simulink model "FSK_MODEM_v2"  (R2021b)
settings: Solver=VariableStepAuto  StartTime=0.0  StopTime=0.05  RelTol=1e-3
values from neighbouring files (symbols this model uses):
  fcarrier = 10000    [run_modem.m]
  fdelta = (fcarrier/100)*50    (= 5000)    [run_modem.m]
libraries: dsparch4 x5, dspsrcs4 x2, commrandsrc3 x1
settings Model: Creator=caccolillo  LastModifiedBy=caccolillo

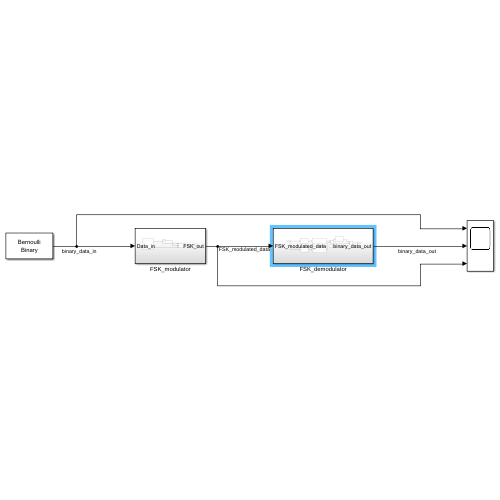
[thumbnail: Simulink's stored preview of the top-level diagram]
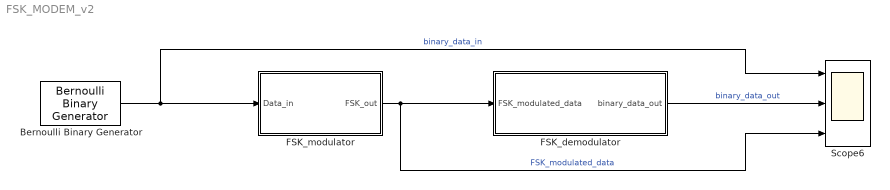
== system FSK_MODEM_v2 ==
  Bernoulli Binary Generator : commrandsrc3/Bernoulli Binary Generator  ProbabilityOfZero=0.5  SeedSource=Auto  Seed=0  SampleTime=20/fcarrier  SamplesPerFrame=1  OutputDataType=double  SimulateUsing=Interpreted execution
  FSK_demodulator : Subsystem
  FSK_modulator : Subsystem
  Scope6 : Scope  NumInputPorts=3
  wires:
  Bernoulli Binary Generator/1 -> FSK_modulator/1(Data_in), Scope6/1  "binary_data_in"
  FSK_demodulator/1(binary_data_out) -> Scope6/2  "binary_data_out"
  FSK_modulator/1(FSK_out) -> Scope6/3, FSK_demodulator/1(FSK_modulated_data)  "FSK_modulated_data"

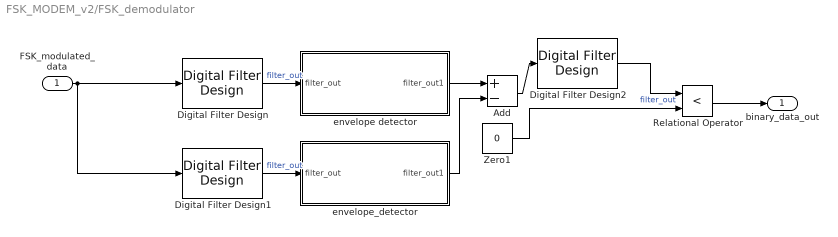
== system FSK_MODEM_v2/FSK_demodulator ==
  FSK_modulated_data : Inport
  Add : Sum  Inputs=+-
  Digital Filter Design : dsparch4/Digital Filter Design  mwdsp_browser_bugfix_var=off
  Digital Filter Design1 : dsparch4/Digital Filter Design  mwdsp_browser_bugfix_var=off
  Digital Filter Design2 : dsparch4/Digital Filter Design  mwdsp_browser_bugfix_var=off
  Relational Operator : RelationalOperator  Operator=<  OutDataTypeStr=boolean  RndMeth=Simplest
  Zero1 : Constant  Value=0  SampleTime=1/(100*fcarrier)
  envelope detector : Subsystem
  envelope_detector : Subsystem
  binary_data_out : Outport
  wires:
  FSK_modulated_data/1 -> Digital Filter Design/1, Digital Filter Design1/1
  Add/1 -> Digital Filter Design2/1
  Digital Filter Design/1 -> envelope detector/1(filter_out)  "filter_out"
  Relational Operator/1 -> binary_data_out/1
  Zero1/1 -> Relational Operator/2
  envelope detector/1(filter_out1) -> Add/1
  envelope_detector/1(filter_out1) -> Add/2
  Digital Filter Design1/1 -> envelope_detector/1(filter_out)  "filter_out"
  Digital Filter Design2/1 -> Relational Operator/1  "filter_out"

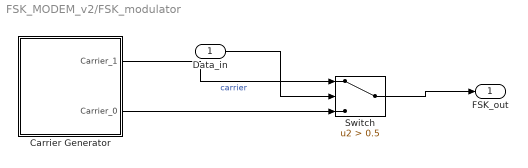
== system FSK_MODEM_v2/FSK_modulator ==
  Data_in : Inport
  "Carrier Generator " : Subsystem
  Switch : Switch  Criteria=u2 > Threshold  Threshold=0.5
  FSK_out : Outport
  wires:
  "Carrier Generator "/1(Carrier_1) -> Switch/1  "carrier"
  "Carrier Generator "/2(Carrier_0) -> Switch/3
  Switch/1 -> FSK_out/1
  Data_in/1 -> Switch/2

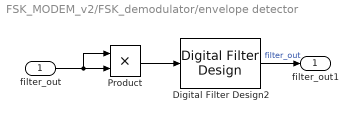
== system FSK_MODEM_v2/FSK_demodulator/envelope detector ==
  filter_out : Inport
  Digital Filter Design2 : dsparch4/Digital Filter Design  mwdsp_browser_bugfix_var=off
  Product : Product
  filter_out1 : Outport
  wires:
  filter_out/1 -> Product/1, Product/2
  Product/1 -> Digital Filter Design2/1
  Digital Filter Design2/1 -> filter_out1/1  "filter_out"

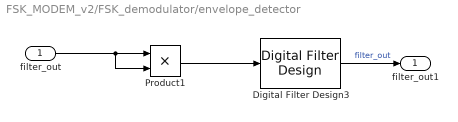
== system FSK_MODEM_v2/FSK_demodulator/envelope_detector ==
  filter_out : Inport
  Digital Filter Design3 : dsparch4/Digital Filter Design  mwdsp_browser_bugfix_var=off
  Product1 : Product
  filter_out1 : Outport
  wires:
  Product1/1 -> Digital Filter Design3/1
  filter_out/1 -> Product1/1, Product1/2
  Digital Filter Design3/1 -> filter_out1/1  "filter_out"

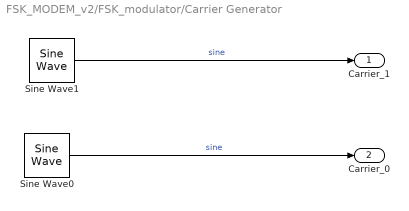
== system FSK_MODEM_v2/FSK_modulator/Carrier Generator  ==
  Sine Wave0 : dspsrcs4/Sine Wave  Amplitude=1  Frequency=fcarrier+fdelta  Phase=0  SampleMode=Discrete  OutComplex=Real  CompMethod=Trigonometric fcn  TableSize=Speed  SampleTime=1/(100*fcarrier)  SamplesPerFrame=1  ResetState=Restart at time zero  OutputFrames=off  dataType=double  wordLen=16  udDataType=sfix(16)  fracBitsMode=Best precision  numFracBits=15  OutDataTypeStr=double  LastOutDataTypeStr=double
  Sine Wave1 : dspsrcs4/Sine Wave  Amplitude=1  Frequency=fcarrier  Phase=0  SampleMode=Discrete  OutComplex=Real  CompMethod=Trigonometric fcn  TableSize=Speed  SampleTime=1/(100*fcarrier)  SamplesPerFrame=1  ResetState=Restart at time zero  OutputFrames=off  dataType=double  wordLen=16  udDataType=sfix(16)  fracBitsMode=Best precision  numFracBits=15  OutDataTypeStr=double  LastOutDataTypeStr=double
  Carrier_1 : Outport  VectorParamsAs1DForOutWhenUnconnected=off
  Carrier_0 : Outport  Port=2  VectorParamsAs1DForOutWhenUnconnected=off
  wires:
  Sine Wave1/1 -> Carrier_1/1  "sine"
  Sine Wave0/1 -> Carrier_0/1  "sine"
